simulink model "SoloModelo"  (R2019b)
settings: Solver=ode1  StartTime=0.0  StopTime=100  FixedStep=ts  RelTol=1e-3
values from neighbouring files (symbols this model uses):
  levitador = imrotate(levitador,90,'bilinear')    [Render.m]
  pelota = imrotate(pelota,90,'bilinear')    [Render.m]
  ts = 0.06    [Render.m]
  ventilador1 = imresize(ventilador1, scale)    [Render.m]
  ventilador2 = imresize(ventilador2, scale)    [Render.m]
undefined symbols (not defined in the file or in its folder): ani12019a, integral, proporcional, referencia
libraries: androiduilib x3, androidaudiovideolib x1
settings Model: Creator=lberm  LastModifiedBy=Hector Augusto Daza
settings OptimizationCC: EnhancedBackFolding=on  PassReuseOutputArgsAs=Individual arguments  ZeroExternalMemoryAtStartup=off  ZeroInternalMemoryAtStartup=off  MaxStackSize=64  OptimizeBlockOrder=speed  DifferentSizesBufferReuse=on  OptimizationCustomize=off  EfficientTunableParamExpr=on
settings DebuggingCC: ParameterTunabilityLossMsg=error  SFMachineParentedDataDiag=error
settings HardwareCC: ProdBitPerPointer=32  ProdBitPerSizeT=32  ProdBitPerPtrDiffT=32  ProdLargestAtomicInteger=Long  ProdLargestAtomicFloat=Double  ProdWordSize=32  ProdHWDeviceType=ARM Compatible->ARM Cortex  UseEmbeddedCoderFeatures=off  UseSimulinkCoderFeatures=off
settings SFSimCC: MATLABDynamicMemAlloc=off  CustomCodeUndefinedFunction=UseInterfaceOnly
settings RTWCC: SystemTargetFile=ert.tlc  HardwareBoard=Android Device  TLCOptions="-aInlineSetEventsForThisBaseRateFcn=TLC_FALSE -aSuppressMultiTaskScheduler=TLC_FALSE  -aRateBasedStepFcn=0"  TemplateMakefile=ert_default_tmf  RTWVerbose=off  Toolchain=Android SDK/NDK Tools
settings CodeAppCC: ForceParamTrailComments=on  IgnoreCustomStorageClasses=off  OperatorAnnotations=on  SimulinkDataObjDesc=on  SFDataObjDesc=on  InsertBlockDesc=on
settings ERTTargetCC: SupportContinuousTime=on  SupportNonInlinedSFcns=on  SupportVariableSizeSignals=on

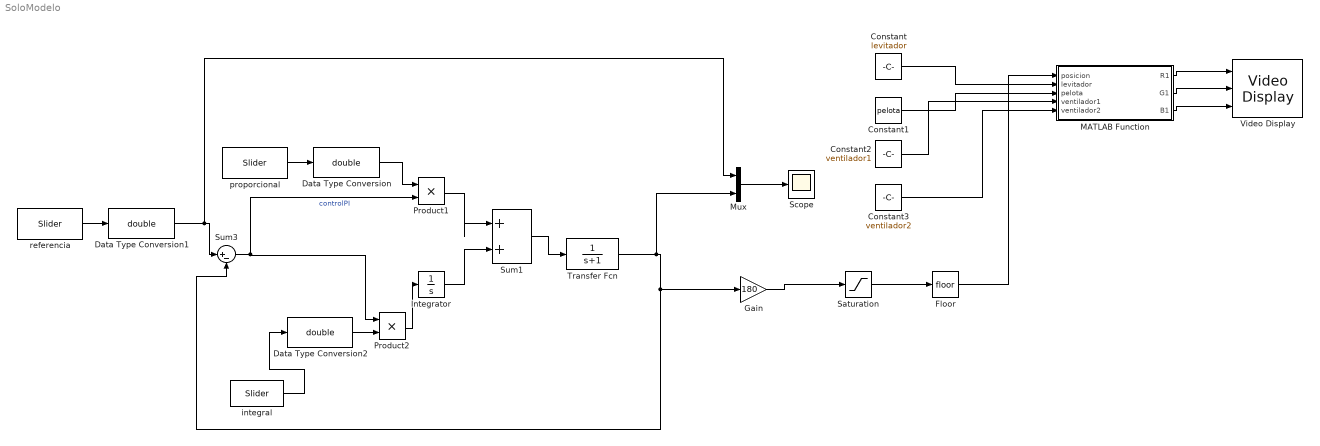
== system SoloModelo ==
  Constant : Constant  Value=levitador  SampleTime=ts
  Constant1 : Constant  Value=pelota  SampleTime=ts
  Constant2 : Constant  Value=ventilador1  SampleTime=ts
  Constant3 : Constant  Value=ventilador2  SampleTime=ts
  Data Type Conversion : DataTypeConversion  OutDataTypeStr=double
  Data Type Conversion1 : DataTypeConversion  OutDataTypeStr=double
  Data Type Conversion2 : DataTypeConversion  OutDataTypeStr=double
  Floor : Rounding
  Gain : Gain  Gain=180
  Integrator : Integrator
  MATLAB Function : MATLAB Function  TreatAsAtomicUnit=on
  Mux : Mux  Inputs=2
  Product1 : Product  OutDataTypeStr=double
  Product2 : Product  OutDataTypeStr=double
  Saturation : Saturate  UpperLimit=180  LowerLimit=0
  Scope : Scope
  Sum1 : Sum  Inputs=|++
  Sum3 : Sum  Inputs=|+-  OutDataTypeStr=double
  Transfer Fcn : TransferFcn  Denominator=[1 1]
  Video Display : androidaudiovideolib/Video Display  BlockPlatform=Android
      settings: SourceProductName=Simulink Support Package for Android Devices  SourceProductBaseCode=ANDROID
  integral : androiduilib/Slider  Min=1  Value=15  Max=20  Resolution=0.1  SliderId=ani12019a/integral  SampleTime=ts  BlockPlatform=Android
      settings: SourceProductName=Simulink Support Package for Android Devices  SourceProductBaseCode=ANDROID
  proporcional : androiduilib/Slider  Min=.01  Value=0.02  Max=2  Resolution=0.01  SliderId=ani12019a/proporcional  SampleTime=ts  BlockPlatform=Android
      settings: SourceProductName=Simulink Support Package for Android Devices  SourceProductBaseCode=ANDROID
  referencia : androiduilib/Slider  Min=0.01  Value=0.5  Max=1  Resolution=0.01  SliderId=ani12019a/referencia  SampleTime=ts  BlockPlatform=Android
      settings: SourceProductName=Simulink Support Package for Android Devices  SourceProductBaseCode=ANDROID
  wires:
  Saturation/1 -> Floor/1
  Product2/1 -> Integrator/1
  Product1/1 -> Sum1/1
  Sum3/1 -> Product1/2, Product2/1  "controlPI"
  Integrator/1 -> Sum1/2
  Sum1/1 -> Transfer Fcn/1
  Transfer Fcn/1 -> Mux/2, Gain/1, Sum3/2
  Mux/1 -> Scope/1
  Gain/1 -> Saturation/1
  proporcional/1 -> Data Type Conversion/1
  Data Type Conversion/1 -> Product1/1
  Data Type Conversion1/1 -> Mux/1, Sum3/1
  referencia/1 -> Data Type Conversion1/1
  integral/1 -> Data Type Conversion2/1
  Data Type Conversion2/1 -> Product2/2
  MATLAB Function/1(R1) -> Video Display/1
  MATLAB Function/2(G1) -> Video Display/2
  MATLAB Function/3(B1) -> Video Display/3
  Floor/1 -> MATLAB Function/1(posicion)
  Constant/1 -> MATLAB Function/2(levitador)
  Constant1/1 -> MATLAB Function/3(pelota)
  Constant2/1 -> MATLAB Function/4(ventilador1)
  Constant3/1 -> MATLAB Function/5(ventilador2)

== matlab function SoloModelo/MATLAB Function ==
  data: posicion input; R1 output; G1 output; B1 output; levitador input; pelota input; ventilador1 input; ventilador2 input
function [R1,G1,B1] = renderLevitador(posicion,levitador,pelota,ventilador1,ventilador2)

if mod((posicion),2)==1
    ventilador=ventilador1;
else
    ventilador=ventilador2;
end

r=ventilador(:,:,1);
g=ventilador(:,:,2);
b=ventilador(:,:,3);
x=220;
y=426;

[n,m]=size(r);
for i=1:n
    for j=1:m
        if r(i,j)<=250 &&  g(i,j)<=250 && b(i,j)<=250
          levitador(i+x,j+y,:)=ventilador(i,j,:);
        end
    end
end

r=pelota(:,:,1);
g=pelota(:,:,2);
b=pelota(:,:,3);

ymax=380;
x=208;

[n,m]=size(r);
for i=1:n
    for j=1:m
        if r(i,j)<=245 &&  g(i,j)<=245 && b(i,j)<=245
          levitador(i+x,j+ymax-posicion,:)=pelota(i,j,:);
        end
    end
end

R1 = uint8(zeros(480,640));
G1 = uint8(zeros(480,640));
B1 = uint8(zeros(480,640));

G1 = levitador(:,:,3);
B1 = levitador(:,:,2);
R1 = levitador(:,:,1);
